simulink model "controlDesignUSV"  (R2021a)
settings: Solver=FixedStepAuto  StartTime=0.0  StopTime=500  FixedStep=SampleTime  RelTol=1e-3
values from neighbouring files (symbols this model uses):
  desideredSpeeds = 0:speedStep:maxSpeed    [identificateUSV.m]
  desideredYawRates = minYawRate:yawRateStep:maxYawRate    [identificateUSV.m]
  FFspeedCommands = interp1([0 speedMeanLevelSteps maxSpeed],                           [0 speedCommandLevelSteps 100],                            desideredSpeeds, 'pchip')    [identificateUSV.m]
  FFyawRateCommands = interp1([0 yawRateMeanLevelStepsFixed minYawRate maxYawRate],                              [0 yawRateCommandLevelStepsFixed -100 100],                              desideredYawRates, 'pchip')    [identificateUSV.m]
  lateralP1D = procest(idData,'P1D')    [identificateUSV.m]
  longitudinalP1D = procest(idData,'P1D')    [identificateUSV.m]
  PIDSampleTime = 0.1    [identificateUSV.m]
  SampleTime = 0.01    [getUSV.m]    (also in identificateUSV.m = mean(diff(USV.time)))
libraries: slctrlblks x2, pid_lib x2, simulink x1
settings Model: EnablePacing=on  PacingRate=5  Creator=frank  LastModifiedBy=frank

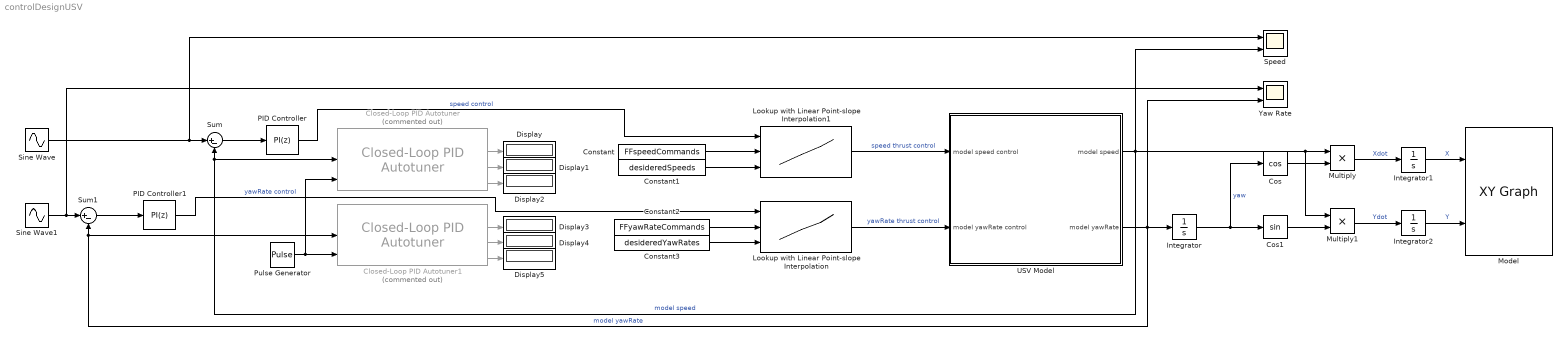
== system controlDesignUSV ==
  Closed-Loop PID Autotuner : slctrlblks/Closed-Loop PID Autotuner  Commented=on  PIDType=PI  PIDForm=Parallel  TimeDomain=discrete-time  DiscreteTs=PIDSampleTime  TuningTs=0.2  UseTuningTs=off  IntegratorFormula=Forward Euler  FilterFormula=Forward Euler  ContinuousTs=0.02  Bandwidth=1  UseExternalWC=off  TargetPM=60  UseExternalPM=off  UseExternalAchievedPM=on  PlantType=Stable  PlantSign=Positive  AmpSine=1  UseExternalAmpSine=off  UseExternalFRD=off  UseExternalU0=off  UseCompanion=off  NotDeployTuningModule=off  UsePLCCoder=off  OutputMode=control action + perturbation  BlockDataType=double  UseConnectedPID=on  blockpath=[]  tunedP=0  tunedI=0  tunedD=0  tunedN=100  tunedPM=0  EstimationWindowSize=3  UseExternalTuningParams=off  OutputChoice=VariantCandD  SingleMultiRateVariant=SingleSamplingRate
      settings: SourceProductBaseCode=SD
  Closed-Loop PID Autotuner1 : slctrlblks/Closed-Loop PID Autotuner  Commented=on  PIDType=PI  PIDForm=Parallel  TimeDomain=discrete-time  DiscreteTs=PIDSampleTime  TuningTs=0.2  UseTuningTs=off  IntegratorFormula=Forward Euler  FilterFormula=Forward Euler  ContinuousTs=0.02  Bandwidth=1  UseExternalWC=off  TargetPM=60  UseExternalPM=off  UseExternalAchievedPM=on  PlantType=Stable  PlantSign=Positive  AmpSine=1  UseExternalAmpSine=off  UseExternalFRD=off  UseExternalU0=off  UseCompanion=off  NotDeployTuningModule=off  UsePLCCoder=off  OutputMode=control action + perturbation  BlockDataType=double  UseConnectedPID=on  blockpath=[]  tunedP=0  tunedI=0  tunedD=0  tunedN=100  tunedPM=0  EstimationWindowSize=3  UseExternalTuningParams=off  OutputChoice=VariantCandD  SingleMultiRateVariant=SingleSamplingRate
      settings: SourceProductBaseCode=SD
  Constant : Constant  Value=FFspeedCommands
  Constant1 : Constant  Value=desideredSpeeds
  Constant2 : Constant  Value=FFyawRateCommands
  Constant3 : Constant  Value=desideredYawRates
  Cos : Trigonometry  Operator=cos
  Cos1 : Trigonometry
  Display{,1..5} (6 alike) : Display
  Integrator : Integrator  WrapState=on
  Integrator1 : Integrator
  Integrator2 : Integrator
  Lookup with Linear Point-slope Interpolation : Lookup_n-D  NumberOfTableDimensions=1  BreakpointsForDimension1Source=Input port  BreakpointsForDimension1=[-5:5]  TableSource=Input port  Table=tanh([-5:5])  InternalRulePriority=Speed  RndMeth=Simplest  InputSameDT=on
      settings: InputPortMap=u0,p221,p5
  Lookup with Linear Point-slope Interpolation1 : Lookup_n-D  NumberOfTableDimensions=1  BreakpointsForDimension1Source=Input port  BreakpointsForDimension1=[-5:5]  TableSource=Input port  Table=tanh([-5:5])  InternalRulePriority=Speed  RndMeth=Simplest  InputSameDT=on
      settings: InputPortMap=u0,p221,p5
  Model : simulink/Sinks/XY Graph  xmin=-40  xmax=15  ymin=-30  ymax=20  st=0.1
  Multiply : Product  Inputs=**
  Multiply1 : Product  Inputs=**
  PID Controller : pid_lib/PID Controller  Controller=PI  Form=Parallel  TimeDomain=Discrete-time  UseExternalTs=off  SampleTime=PIDSampleTime  IntegratorMethod=Forward Euler  FilterMethod=Forward Euler  ControllerParametersSource=internal  P=4.8991  I=1.7911  D=0  UseFilter=on  N=100  TunerSelectOption=Transfer Function Based (PID Tuner App)  InitialConditionSource=internal  InitialConditionForIntegrator=0  InitialConditionForFilter=0  DifferentiatorICPrevScaledInput=0  ExternalReset=none  TrackingMode=off  Kt=1  LimitOutput=on  SatLimitsSource=internal  UpperSaturationLimit=80  LowerSaturationLimit=0  LinearizeAsGain=on  AntiWindupMode=clamping  Kb=1  POutMin=[]  POutMax=[]  IOutMin=[]  IOutMax=[]  DOutMin=[]  DOutMax=[]  NOutMin=[]  NOutMax=[]  SumOutMin=[]  SumOutMax=[]  SaturationOutMin=[]  SaturationOutMax=[]  PParamMin=[]  PParamMax=[]  IParamMin=[]  IParamMax=[]  DParamMin=[]  DParamMax=[]  NParamMin=[]  NParamMax=[]  KbParamMin=[]  KbParamMax=[]  KtParamMin=[]  KtParamMax=[]  KbOutMin=[]  KbOutMax=[]  KtOutMin=[]  KtOutMax=[]  IntegratorOutMin=[]  IntegratorOutMax=[]  FilterOutMin=[]  FilterOutMax=[]  SumI1OutMin=[]  SumI1OutMax=[]  SumI2OutMin=[]  SumI2OutMax=[]  SumI3OutMin=[]  SumI3OutMax=[]  SumI4OutMin=[]  SumI4OutMax=[]  SumDOutMin=[]  SumDOutMax=[]  DifferentiatorOutMin=[]  DifferentiatorOutMax=[]  FilterDiffOutCoefMin=[]  FilterDiffOutCoefMax=[]  ReciprocalOutMin=[]  ReciprocalOutMax=[]  SumDenOutMin=[]  SumDenOutMax=[]  SumNumOutMin=[]  SumNumOutMax=[]  DivideOutMin=[]  DivideOutMax=[]  UdiffTsProdOutMin=[]  UdiffTsProdOutMax=[]  NTsProdOutMin=[]  NTsProdOutMax=[]  UintegralTsProdOutMin=[]  UintegralTsProdOutMax=[]  UngainTsProdOutMin=[]  UngainTsProdOutMax=[]  IntegratorContinuousStateAttributes=''  IntegratorStateMustResolveToSignalObject=off  IntegratorRTWStateStorageClass=Auto  FilterContinuousStateAttributes=''  FilterStateMustResolveToSignalObject=off  FilterRTWStateStorageClass=Auto  ParallelPVariant=InternalParameters  IdealPVariant=Disabled  IVariant=InternalParameters  DVariant=Disabled  IntegratorVariant=Discrete  SatVariant=Enabled  AWVariant=DiscClampingParallel  PCopyVariant=Disabled  TRVariant=Disabled  FdbkBlocksVariant=Forward  IdealPFdbkVariant=Disabled  SatFdbkVariant=Disabled  DerivativeFilterVariant=Disabled  NVariant=Disabled  NCopyVariant=Disabled_SignalSpec  FilterICVariant=Disabled  IntegratorICVariant=InternalICs  ExternalResetVariant=Disabled  TRSumVariant=Passthrough  SumFdbkVariant=Disabled  SumVariant=Sum_PI  TsampFilterVariant=InternalTs  TsampNgainVariant=Passthrough  TsampIntegralVariant=Passthrough  ExternalSaturationOutDataTypeStr=Inherit: Same as second input
  PID Controller1 : pid_lib/PID Controller  Controller=PI  Form=Parallel  TimeDomain=Discrete-time  UseExternalTs=off  SampleTime=PIDSampleTime  IntegratorMethod=Forward Euler  FilterMethod=Forward Euler  ControllerParametersSource=internal  P=4.8246  I=19.0144  D=0  UseFilter=on  N=100  TunerSelectOption=Transfer Function Based (PID Tuner App)  InitialConditionSource=internal  InitialConditionForIntegrator=0  InitialConditionForFilter=0  DifferentiatorICPrevScaledInput=0  ExternalReset=none  TrackingMode=off  Kt=1  LimitOutput=on  SatLimitsSource=internal  UpperSaturationLimit=60  LowerSaturationLimit=-60  LinearizeAsGain=on  AntiWindupMode=clamping  Kb=1  POutMin=[]  POutMax=[]  IOutMin=[]  IOutMax=[]  DOutMin=[]  DOutMax=[]  NOutMin=[]  NOutMax=[]  SumOutMin=[]  SumOutMax=[]  SaturationOutMin=[]  SaturationOutMax=[]  PParamMin=[]  PParamMax=[]  IParamMin=[]  IParamMax=[]  DParamMin=[]  DParamMax=[]  NParamMin=[]  NParamMax=[]  KbParamMin=[]  KbParamMax=[]  KtParamMin=[]  KtParamMax=[]  KbOutMin=[]  KbOutMax=[]  KtOutMin=[]  KtOutMax=[]  IntegratorOutMin=[]  IntegratorOutMax=[]  FilterOutMin=[]  FilterOutMax=[]  SumI1OutMin=[]  SumI1OutMax=[]  SumI2OutMin=[]  SumI2OutMax=[]  SumI3OutMin=[]  SumI3OutMax=[]  SumI4OutMin=[]  SumI4OutMax=[]  SumDOutMin=[]  SumDOutMax=[]  DifferentiatorOutMin=[]  DifferentiatorOutMax=[]  FilterDiffOutCoefMin=[]  FilterDiffOutCoefMax=[]  ReciprocalOutMin=[]  ReciprocalOutMax=[]  SumDenOutMin=[]  SumDenOutMax=[]  SumNumOutMin=[]  SumNumOutMax=[]  DivideOutMin=[]  DivideOutMax=[]  UdiffTsProdOutMin=[]  UdiffTsProdOutMax=[]  NTsProdOutMin=[]  NTsProdOutMax=[]  UintegralTsProdOutMin=[]  UintegralTsProdOutMax=[]  UngainTsProdOutMin=[]  UngainTsProdOutMax=[]  IntegratorContinuousStateAttributes=''  IntegratorStateMustResolveToSignalObject=off  IntegratorRTWStateStorageClass=Auto  FilterContinuousStateAttributes=''  FilterStateMustResolveToSignalObject=off  FilterRTWStateStorageClass=Auto  ParallelPVariant=InternalParameters  IdealPVariant=Disabled  IVariant=InternalParameters  DVariant=Disabled  IntegratorVariant=Discrete  SatVariant=Enabled  AWVariant=DiscClampingParallel  PCopyVariant=Disabled  TRVariant=Disabled  FdbkBlocksVariant=Forward  IdealPFdbkVariant=Disabled  SatFdbkVariant=Disabled  DerivativeFilterVariant=Disabled  NVariant=Disabled  NCopyVariant=Disabled_SignalSpec  FilterICVariant=Disabled  IntegratorICVariant=InternalICs  ExternalResetVariant=Disabled  TRSumVariant=Passthrough  SumFdbkVariant=Disabled  SumVariant=Sum_PI  TsampFilterVariant=InternalTs  TsampNgainVariant=Passthrough  TsampIntegralVariant=Passthrough  ExternalSaturationOutDataTypeStr=Inherit: Same as second input
  Pulse Generator : DiscretePulseGenerator  PulseType=Time based  Period=500  PulseWidth=80  PhaseDelay=10
  Sine Wave : Sin  Amplitude=1.5  Bias=1.5  Frequency=0.3  SampleTime=SampleTime
  Sine Wave1 : Sin  Amplitude=0.5  Frequency=0.5  SampleTime=SampleTime
  Speed : Scope  NumInputPorts=2
  Sum : Sum  Inputs=|+-
  Sum1 : Sum  Inputs=|+-
  USV Model : Subsystem
  Yaw Rate : Scope  NumInputPorts=2
  wires:
  Integrator/1 -> Cos1/1, Cos/1  "yaw"
  Cos/1 -> Multiply/2
  Cos1/1 -> Multiply1/2
  Multiply/1 -> Integrator1/1  "Xdot"
  Multiply1/1 -> Integrator2/1  "Ydot"
  Integrator1/1 -> Model/1  "X"
  Integrator2/1 -> Model/2  "Y"
  Lookup with Linear Point-slope Interpolation1/1 -> USV Model/1(model speed control)  "speed thrust control"
  Lookup with Linear Point-slope Interpolation/1 -> USV Model/2(model yawRate control)  "yawRate thrust control"
  USV Model/2(model yawRate) -> Closed-Loop PID Autotuner1/2, Sum1/2, Integrator/1, Yaw Rate/2  "model yawRate"
  USV Model/1(model speed) -> Closed-Loop PID Autotuner/2, Sum/2, Multiply1/1, Multiply/1, Speed/2  "model speed"
  Constant2/1 -> Lookup with Linear Point-slope Interpolation/2
  Constant1/1 -> Lookup with Linear Point-slope Interpolation1/3
  Constant/1 -> Lookup with Linear Point-slope Interpolation1/2
  Constant3/1 -> Lookup with Linear Point-slope Interpolation/3
  PID Controller/1 -> Lookup with Linear Point-slope Interpolation1/1  "speed control"
  PID Controller1/1 -> Lookup with Linear Point-slope Interpolation/1  "yawRate control"
  Closed-Loop PID Autotuner/2 -> Display/1
  Closed-Loop PID Autotuner/3 -> Display1/1
  Closed-Loop PID Autotuner/4 -> Display2/1
  Closed-Loop PID Autotuner1/4 -> Display5/1
  Closed-Loop PID Autotuner1/3 -> Display4/1
  Closed-Loop PID Autotuner1/2 -> Display3/1
  Sum/1 -> PID Controller/1
  Sum1/1 -> PID Controller1/1
  Pulse Generator/1 -> Closed-Loop PID Autotuner1/3, Closed-Loop PID Autotuner/3
  Sine Wave/1 -> Speed/1, Sum/1
  Sine Wave1/1 -> Yaw Rate/1, Sum1/1

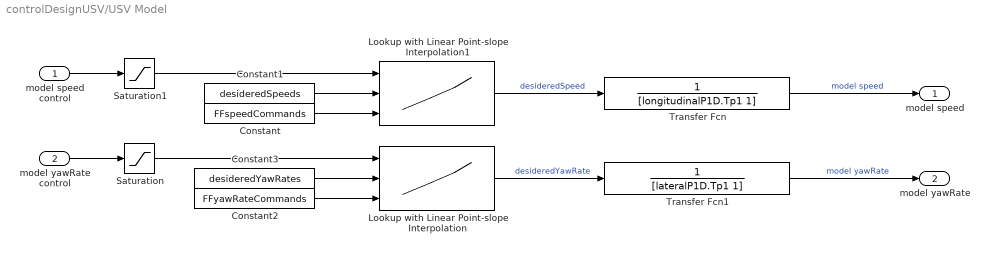
== system controlDesignUSV/USV Model ==
  model speed control : Inport
  model yawRate control : Inport  Port=2
  Constant : Constant  Value=FFspeedCommands
  Constant1 : Constant  Value=desideredSpeeds
  Constant2 : Constant  Value=FFyawRateCommands
  Constant3 : Constant  Value=desideredYawRates
  Lookup with Linear Point-slope Interpolation : Lookup_n-D  NumberOfTableDimensions=1  BreakpointsForDimension1Source=Input port  BreakpointsForDimension1=[-5:5]  TableSource=Input port  Table=tanh([-5:5])  InternalRulePriority=Speed  RndMeth=Simplest  InputSameDT=on
      settings: InputPortMap=u0,p221,p5
  Lookup with Linear Point-slope Interpolation1 : Lookup_n-D  NumberOfTableDimensions=1  BreakpointsForDimension1Source=Input port  BreakpointsForDimension1=[-5:5]  TableSource=Input port  Table=tanh([-5:5])  InternalRulePriority=Speed  RndMeth=Simplest  InputSameDT=on
      settings: InputPortMap=u0,p221,p5
  Saturation : Saturate  UpperLimit=60  LowerLimit=-60
  Saturation1 : Saturate  UpperLimit=80  LowerLimit=0
  Transfer Fcn : TransferFcn  Denominator=[longitudinalP1D.Tp1 1]
  Transfer Fcn1 : TransferFcn  Denominator=[lateralP1D.Tp1 1]
  model speed : Outport
  model yawRate : Outport  Port=2
  wires:
  Lookup with Linear Point-slope Interpolation/1 -> Transfer Fcn1/1  "desideredYawRate"
  Constant3/1 -> Lookup with Linear Point-slope Interpolation/2
  Constant1/1 -> Lookup with Linear Point-slope Interpolation1/2
  Constant2/1 -> Lookup with Linear Point-slope Interpolation/3
  Transfer Fcn/1 -> model speed/1  "model speed"
  Lookup with Linear Point-slope Interpolation1/1 -> Transfer Fcn/1  "desideredSpeed"
  Constant/1 -> Lookup with Linear Point-slope Interpolation1/3
  model speed control/1 -> Saturation1/1
  model yawRate control/1 -> Saturation/1
  Transfer Fcn1/1 -> model yawRate/1  "model yawRate"
  Saturation/1 -> Lookup with Linear Point-slope Interpolation/1
  Saturation1/1 -> Lookup with Linear Point-slope Interpolation1/1
